simulink model "heat_temp"  (R2024b)
settings: Solver=VariableStepAuto  StartTime=0.0  StopTime=10.0  RelTol=1e-3
settings Model: Creator=Ajay1  LastModifiedBy=Ajay1

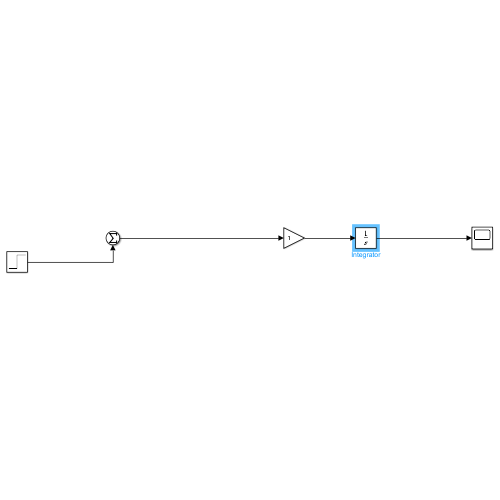
[thumbnail: Simulink's stored preview of the top-level diagram]
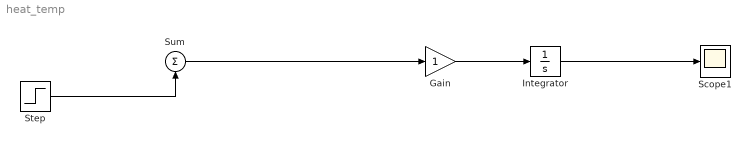
== system heat_temp ==
  Gain : Gain
  Integrator : Integrator  InitialCondition=1
  Scope1 : Scope
  Step : Step  After=5  SampleTime=0
  Sum : Sum  Inputs=|+
  wires:
  Step/1 -> Sum/1
  Gain/1 -> Integrator/1
  Sum/1 -> Gain/1
  Integrator/1 -> Scope1/1
